simulink model "SistemaFunivia"  (R2023b)
settings: Solver=VariableStepAuto  StartTime=0.0  StopTime=10  FixedStep=1e-5  MaxStep=2e-5
values from neighbouring files (symbols this model uses):
  dq_0 = [0; 0]    [Parametri.m]
  encoder_params = [r, encoder_accuracy, encoder_resolution, encoder_sample_rates]    [Parametri.m]
  encoder_resolution = 2*pi/1200    (= 0.00523598775598)    [Parametri.m]
  F_0 = +200    (= 200)    [Parametri.m]
  L = 2.2    [Parametri.m]
  l = L - 1.2    (= 1)    [Parametri.m]
  laserd1_params = [laserd1_sample_rates, laserd1_resolution, laserd1_accuracy]    [Parametri.m]
  laserD_params = [laserD_sample_rates, laserD_resolution, laserD_accuracy]    [Parametri.m]
  min_sample_rates = max(sample_rates)    [Parametri.m]
  params = [m, c_a, J, L, l, h, r, g]    [Parametri.m]
  q_0 = [0; 0]    [Parametri.m]
  R_k = diag([(laserD_accuracy/1000)^2, (laserd1_accuracy/1000)^2, (encoder_accuracy/encoder_sample_rates)^2])    [Parametri.m]
libraries: simulink x4, dspswit3 x1, embmathops x1
settings Model: Creator=lucag  LastModifiedBy=lucag

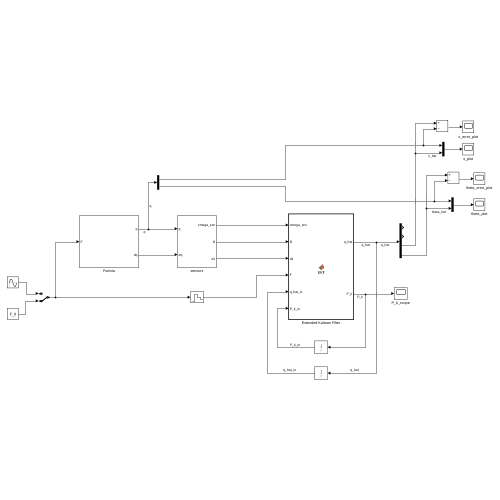
[thumbnail: Simulink's stored preview of the top-level diagram]
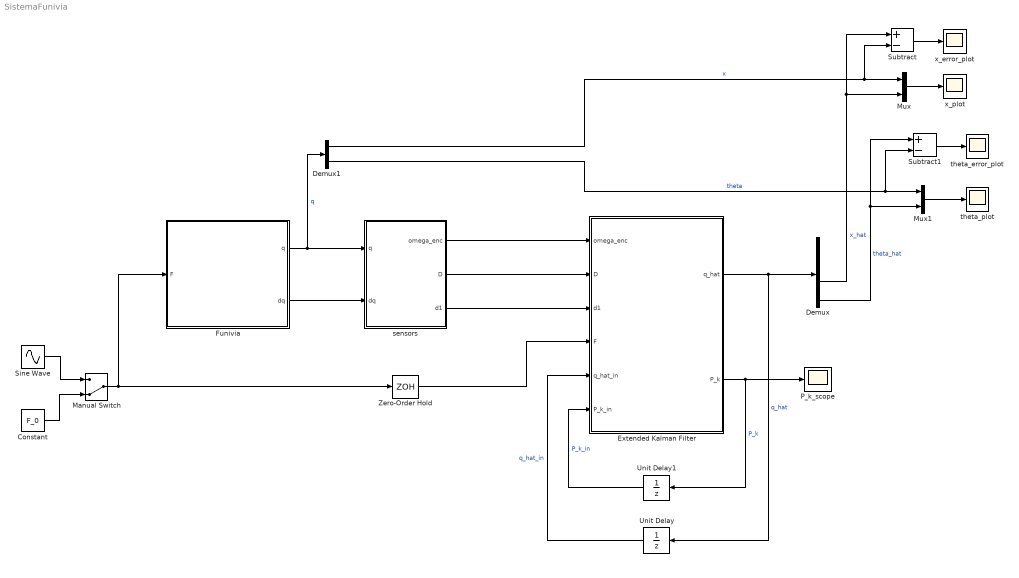
== system SistemaFunivia ==
  Constant : Constant  Value=F_0
  Demux : Demux
  Demux1 : Demux  Outputs=2
  Extended Kalman Filter : MATLAB Function  TreatAsAtomicUnit=on
  Funivia : Subsystem
  Manual Switch : ManualSwitch  CurrentSetting=0
  Mux : Mux  Inputs=2
  Mux1 : Mux  Inputs=2
  P_k_scope : Scope
  Sine Wave : Sin  Amplitude=F_0  SampleTime=0
  Subtract : Sum  Inputs=+-
  Subtract1 : Sum  Inputs=+-
  Unit Delay : UnitDelay  InitialCondition=zeros(4,1)  SampleTime=-1  HasFrameUpgradeWarning=on
  Unit Delay1 : UnitDelay  InitialCondition=eye(4)  SampleTime=-1  HasFrameUpgradeWarning=on
  Zero-Order Hold : ZeroOrderHold  SampleTime=min_sample_rates
  sensors : Subsystem
  theta_error_plot : Scope
  theta_plot : Scope
  x_error_plot : Scope
  x_plot : Scope
  wires:
  Constant/1 -> Manual Switch/2
  Sine Wave/1 -> Manual Switch/1
  Manual Switch/1 -> Funivia/1(F), Zero-Order Hold/1
  Funivia/1(q) -> Demux1/1, sensors/1(q)  "q"
  Funivia/2(dq) -> sensors/2(dq)
  sensors/1(omega_enc) -> Extended Kalman Filter/1(omega_enc)
  sensors/2(D) -> Extended Kalman Filter/2(D)
  sensors/3(d1) -> Extended Kalman Filter/3(d1)
  Zero-Order Hold/1 -> Extended Kalman Filter/4(F)
  Extended Kalman Filter/1(q_hat) -> Unit Delay/1, Demux/1  "q_hat"
  Extended Kalman Filter/2(P_k) -> Unit Delay1/1, P_k_scope/1  "P_k"
  Unit Delay1/1 -> Extended Kalman Filter/6(P_k_in)  "P_k_in"
  Unit Delay/1 -> Extended Kalman Filter/5(q_hat_in)  "q_hat_in"
  Demux1/1 -> Subtract/2, Mux/1  "x"
  Demux/3 -> Subtract/1, Mux/2  "x_hat"
  Demux1/2 -> Subtract1/2, Mux1/1  "theta"
  Demux/4 -> Mux1/2, Subtract1/1  "theta_hat"
  Mux/1 -> x_plot/1
  Mux1/1 -> theta_plot/1
  Subtract/1 -> x_error_plot/1
  Subtract1/1 -> theta_error_plot/1

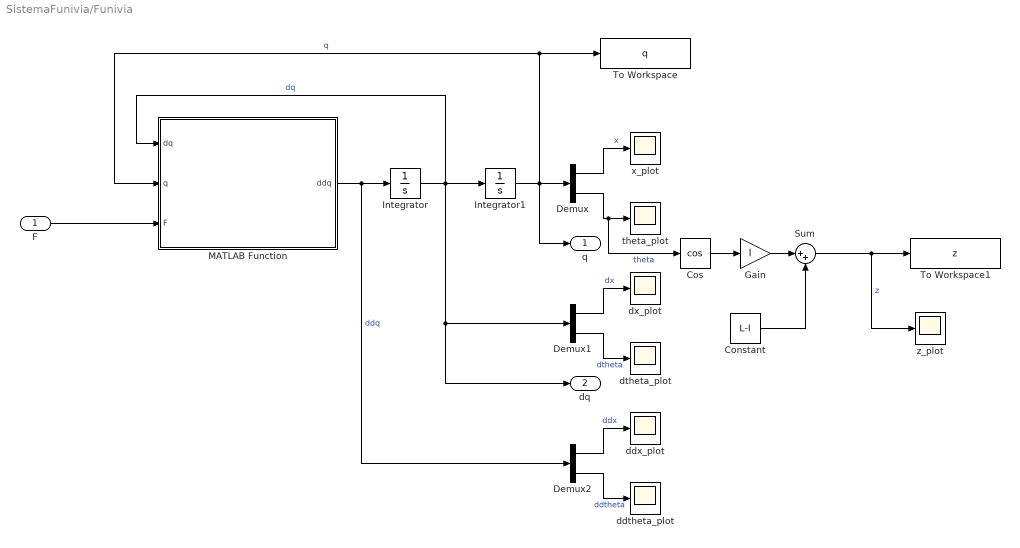
== system SistemaFunivia/Funivia ==
  F : Inport
  Constant : Constant  Value=L-l
  Cos : Trigonometry  Operator=cos
  Demux : Demux  Outputs=2
  Demux1 : Demux  Outputs=2
  Demux2 : Demux  Outputs=2
  Gain : Gain  Gain=l
  Integrator : Integrator  InitialCondition=dq_0
  Integrator1 : Integrator  InitialCondition=q_0
  MATLAB Function : MATLAB Function  TreatAsAtomicUnit=on
  Sum : Sum  Inputs=|++
  To Workspace : ToWorkspace  VariableName=q  SaveFormat=Timeseries  SampleTime=-1
  To Workspace1 : ToWorkspace  VariableName=z  SaveFormat=Timeseries  SampleTime=-1
  ddtheta_plot : Scope
  ddx_plot : Scope
  dtheta_plot : Scope
  dx_plot : Scope
  theta_plot : Scope
  x_plot : Scope
  z_plot : Scope
  q : Outport
  dq : Outport  Port=2
  wires:
  Demux/1 -> x_plot/1  "x"
  MATLAB Function/1(ddq) -> Demux2/1, Integrator/1  "ddq"
  Demux2/1 -> ddx_plot/1  "ddx"
  Integrator1/1 -> q/1, Demux/1, To Workspace/1, MATLAB Function/2(q)  "q"
  Integrator/1 -> dq/1, Demux1/1, MATLAB Function/1(dq), Integrator1/1  "dq"
  Demux2/2 -> ddtheta_plot/1  "ddtheta"
  Demux1/2 -> dtheta_plot/1  "dtheta"
  Demux/2 -> Cos/1, theta_plot/1  "theta"
  Demux1/1 -> dx_plot/1  "dx"
  F/1 -> MATLAB Function/3(F)
  Cos/1 -> Gain/1
  Gain/1 -> Sum/1
  Sum/1 -> z_plot/1, To Workspace1/1  "z"
  Constant/1 -> Sum/2

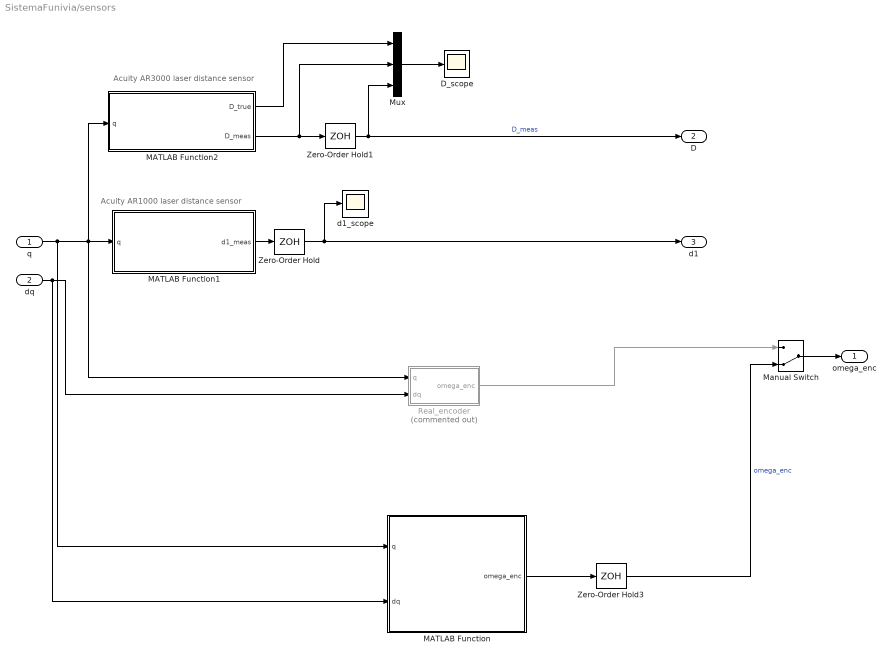
== system SistemaFunivia/sensors ==
  note: Acuity AR1000 laser distance sensor
  note: Acuity AR3000 laser distance sensor
  q : Inport
  dq : Inport  Port=2
  D_scope : Scope
  MATLAB Function : MATLAB Function  TreatAsAtomicUnit=on
  MATLAB Function1 : MATLAB Function  TreatAsAtomicUnit=on
  MATLAB Function2 : MATLAB Function  TreatAsAtomicUnit=on  SystemSampleTime=1/100
  Manual Switch : ManualSwitch  CurrentSetting=0
  Mux : Mux  Inputs=3
  Real_encoder : Subsystem  Commented=on
  Zero-Order Hold : ZeroOrderHold  SampleTime=min_sample_rates
  Zero-Order Hold1 : ZeroOrderHold  SampleTime=min_sample_rates
  Zero-Order Hold3 : ZeroOrderHold  SampleTime=min_sample_rates
  d1_scope : Scope
  omega_enc : Outport
  D : Outport  Port=2
  d1 : Outport  Port=3
  wires:
  Zero-Order Hold/1 -> d1/1, d1_scope/1
  Zero-Order Hold1/1 -> D/1, Mux/3  "D_meas"
  Mux/1 -> D_scope/1
  q/1 -> MATLAB Function/1(q), Real_encoder/1(q), MATLAB Function2/1(q), MATLAB Function1/1(q)
  MATLAB Function2/2(D_meas) -> Mux/2, Zero-Order Hold1/1
  MATLAB Function2/1(D_true) -> Mux/1
  MATLAB Function1/1(d1_meas) -> Zero-Order Hold/1
  dq/1 -> Real_encoder/2(dq), MATLAB Function/2(dq)
  Manual Switch/1 -> omega_enc/1
  MATLAB Function/1(omega_enc) -> Zero-Order Hold3/1
  Zero-Order Hold3/1 -> Manual Switch/2  "omega_enc"
  Real_encoder/1(omega_enc) -> Manual Switch/1

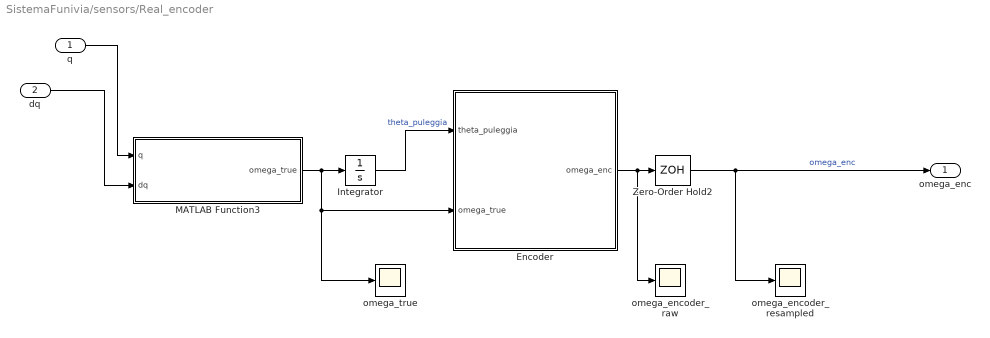
== system SistemaFunivia/sensors/Real_encoder ==
  q : Inport
  dq : Inport  Port=2
  Encoder : Subsystem
  Integrator : Integrator
  MATLAB Function3 : MATLAB Function  TreatAsAtomicUnit=on
  Zero-Order Hold2 : ZeroOrderHold  SampleTime=min_sample_rates
  omega_encoder_raw : Scope
  omega_encoder_resampled : Scope
  omega_true : Scope
  omega_enc : Outport
  wires:
  q/1 -> MATLAB Function3/1(q)
  Encoder/1(omega_enc) -> omega_encoder_raw/1, Zero-Order Hold2/1
  MATLAB Function3/1(omega_true) -> Encoder/2(omega_true), omega_true/1, Integrator/1
  dq/1 -> MATLAB Function3/2(dq)
  Integrator/1 -> Encoder/1(theta_puleggia)  "theta_puleggia"
  Zero-Order Hold2/1 -> omega_enc/1, omega_encoder_resampled/1  "omega_enc"

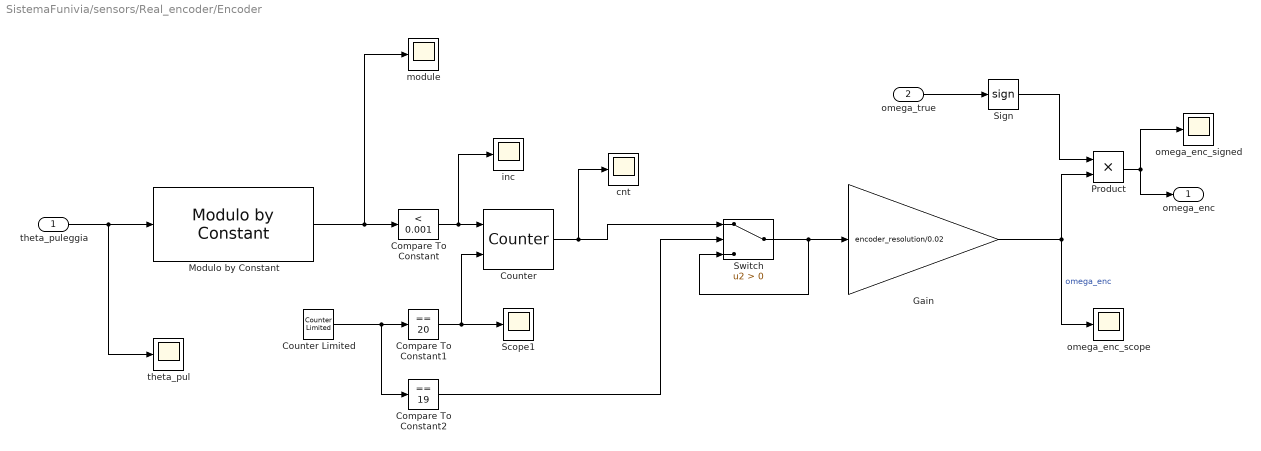
== system SistemaFunivia/sensors/Real_encoder/Encoder ==
  theta_puleggia : Inport
  omega_true : Inport  Port=2
  Compare To Constant : simulink/Logic and Bit Operations/Compare To Constant  relop=<  const=0.001  OutDataTypeStr=boolean
  Compare To Constant1 : simulink/Logic and Bit Operations/Compare To Constant  relop===  const=20  OutDataTypeStr=boolean
  Compare To Constant2 : simulink/Logic and Bit Operations/Compare To Constant  relop===  const=19  OutDataTypeStr=boolean
  Counter : dspswit3/Counter  Direction=Up  CountEvent=Rising edge  CounterSize=User defined  MaxCount=65535  InitialCount=0  Output=Count  HitValue=32  ResetInput=on  SamplesPerFrame=1  Ts=1  CntDtype=double  HitDtype=Logical
  Counter Limited : simulink/Sources/Counter Limited  uplimit=20  tsamp=0.001
  Gain : Gain  Gain=encoder_resolution/0.02
  Modulo by Constant : embmathops/Modulo by Constant  Denominator=encoder_resolution  SimulateUsing=Code generation
      settings: LibrarySourceBlock=embeddedMathLib/Modulo by Constant
  Product : Product
  Scope1 : Scope
  Sign : Signum
  Switch : Switch  Criteria=u2 > Threshold  SaturateOnIntegerOverflow=off  InputSameDT=off
  cnt : Scope
  inc : Scope
  module : Scope
  omega_enc_scope : Scope
  omega_enc_signed : Scope
  theta_pul : Scope
  omega_enc : Outport
  wires:
  Counter/1 -> cnt/1, Switch/1
  Switch/1 -> Switch/3, Gain/1
  Modulo by Constant/1 -> module/1, Compare To Constant/1
  Counter Limited/1 -> Compare To Constant2/1, Compare To Constant1/1
  Compare To Constant1/1 -> Scope1/1, Counter/2
  Gain/1 -> Product/2, omega_enc_scope/1  "omega_enc"
  Compare To Constant2/1 -> Switch/2
  Compare To Constant/1 -> inc/1, Counter/1
  theta_puleggia/1 -> Modulo by Constant/1, theta_pul/1
  omega_true/1 -> Sign/1
  Product/1 -> omega_enc_signed/1, omega_enc/1
  Sign/1 -> Product/1

== matlab function SistemaFunivia/sensors/MATLAB Function2 ==
  settings: updateMethod=DISCRETE  sampleTime=laserD_sample_rates
  data: D_true output; D_meas output; q input; params parameter; laserD_params parameter
function [D_true, D_meas] = Sensore_Laser_D(q, params, laserD_params)
    laserD_accuracy = laserD_params(3); %[mm]
    l = params(5)*1000; %[mm]
    r = params(7)*1000; %[mm]

    x = q(1)*1000; %[mm]
    theta = q(2);

    D_true = x + (l+r)*sin(theta);  % [mm]
    noise = normrnd(0, laserD_accuracy/3);  %considering that +- 3*dev_std is the 95perc confidence

    D_meas = D_true + noise;   % convert the data params from meters to mm, because the noise is in mm
    D_meas = round(D_meas)/1000;
end

== matlab function SistemaFunivia/Funivia/MATLAB Function ==
  data: dq input; ddq output; q input; F input; params parameter
    function ddq = ModelloDinamicoFunivia(dq, q, F, params)
    
    % Variabili di Stato %
    dx = dq(1);
    dtheta = dq(2);

    x = q(1);
    theta = q(2);
   
    % Parametri fisici %
    m = params(1);
    c_a = params(2);
    J = params(3);

    L = params(4);
    l = params(5);
    h = params(6);
    r = params(7);

    g = params(8);

    % Equazioni del modello fisico %
    ddx = -c_a/m * (dx - (l + r)*dtheta*cos(theta)) + F/m;
    ddtheta = -m*g*(l + r)/J * sin(theta) + c_a*(l + r)/J * (dx - (l + r)*dtheta*cos(theta)) - F*L/J * cos(theta);

    ddq = [ddx; ddtheta];

end

== matlab function SistemaFunivia/sensors/MATLAB Function1 ==
  settings: updateMethod=DISCRETE  sampleTime=laserd1_sample_rates
  data: d1_meas output; q input; params parameter; laserd1_params parameter
function d1_meas = Sensore_Laser_d1(q, params, laserd1_params)
    
    L = params(4);
    h = params(6);

    laser_accuracy = laserd1_params(3);

    theta = q(2);
    
    d1_true = (L + h) * 1000 * cos(theta);    % [mm]
    noise = normrnd(0, laser_accuracy/3);

    d1_meas = d1_true + noise;
    d1_meas = round(d1_meas) / 1000;    % to meters

end

== matlab function SistemaFunivia/sensors/Real_encoder/MATLAB Function3 ==
  settings: updateMethod=CONTINUOUS  sampleTime=encoder_sample_rates
  data: omega_true output; q input; params parameter; encoder_params parameter; dq input
function omega_true = puleggia(q, params, encoder_params, dq)
    
    l = params(5); % [m]
    r = encoder_params(1); % [m]

    theta = q(2); % [rad]

    dx = dq(1); % [m/s]
    dtheta = dq(2); % [rad/s]

    v_c = dx - l*dtheta*cos(theta); %equation
    
    omega_true = v_c/r;    % [rad/s]
    % noise = normrnd(0, encoder_accuracy/3);
    % 
    % omega_meas = omega_true + noise;
    % omega = round(omega_meas);

end

== matlab function SistemaFunivia/Extended Kalman Filter ==
  settings: updateMethod=DISCRETE  sampleTime=min_sample_rates
  data: omega_enc input; D input; d1 input; params parameter; encoder_params parameter; F input; min_sample_rates parameter; q_hat output; P_k output; R_k parameter; q_hat_in input; P_k_in input
                                                             function [q_hat, P_k] = EKF(omega_enc, D, d1, params, encoder_params, F, min_sample_rates, R_k, q_hat_in, P_k_in)

m = params(1);
c_a = params(2);
J = params(3);

L = params(4);
l = params(5);
h = params(6);

g = params(7);

r = encoder_params(1);

q1 = q_hat_in(1);
q2 = q_hat_in(2);
q3 = q_hat_in(3);
q4 = q_hat_in(4);

F_k = [-c_a/m,          (c_a/m)*(l+r)*cos(q4),      0,      -(c_a/m)*(l+r)*q2*sin(q4);
        c_a*(l+r)/J,    -(c_a*(l+r)^2/J)*cos(q4),   0,      -(m*g*(l+r)/J)*cos(q4) + (c_a*(l+r)^2/J)*q2*sin(q4) + F*(L/J)*sin(q4);
        1,              0,                          0,      0;
        0,              1,                          0,      0];
F_k = min_sample_rates .* F_k + eye(4);    % from TC to TD q_dot => (q_k+1 - q_k)/dT = F_k * q_k

D_k = [1/m;
      -(L/J)*cos(q4);
      0;
      0];
D_k = min_sample_rates .* D_k;

y_k = [D;
       d1;
       omega_enc];

H_k = [0,           0,                      1,      (l+h)*cos(q4);
       0,           0,                      0,      -(L+h)*sin(q4);
       1/r,         -(l/r)*cos(q4),         0,      (l/r)*q2*sin(q4)];


M_k = eye(3);   %hyp: Gaussian noise equally distributed on each sensor measurements

dev_std = 2;
Q_k = dev_std^2 .* eye(4);

%% prediction
P_k = F_k * P_k_in * F_k' + D_k' * Q_k * D_k;

input_noise = 0;
q_hat = F_k * q_hat_in + (F + input_noise).*D_k;

%% correction
h_k = [ q3 + (l+h)*sin(q4);
        (L+h)*cos(q4);
        (1/r)*(q1 - l*q2*cos(q4))];

e_k = y_k - h_k;
S_k = H_k * P_k_in * H_k' + M_k * R_k * M_k';
L_k = P_k_in * H_k' * S_k^(-1);

q_hat = q_hat + L_k * e_k;
% P_k = P_k - L_k * S_k * L_k';
P_k = (eye(4) - L_k * H_k)*P_k*(eye(4) - L_k*H_k)' + L_k * M_k * R_k * M_k' * L_k';

end

== matlab function SistemaFunivia/sensors/MATLAB Function ==
  settings: updateMethod=DISCRETE  sampleTime=encoder_sample_rates
  data: q input; dq input; omega_enc output; params parameter; encoder_params parameter
function omega_enc = encoder(q, dq, params, encoder_params)
    l = params(5);
    r = encoder_params(1);
    encoder_accuracy = encoder_params(2);
    encoder_sample_rates = encoder_params(4);

    theta = q(2);
    dtheta = dq(2);
    dx = dq(1);
    
    omega_true = (dx - (l+r)*dtheta*cos(theta))/r;    % [rad/s]
    noise = normrnd(0, encoder_accuracy/(encoder_sample_rates * 3));

    omega_enc = omega_true + noise;

end
